simulink model "K_linearLUB"  (R2016a)
settings: Solver=VariableStepAuto  StartTime=0.0  StopTime=1000.0  RelTol=1e-3
undefined symbols (not defined in the file): A, AKL, B, BL, C, CO, D, DO, K, X0
settings Model: Creator=kp  LastModifiedBy=kp

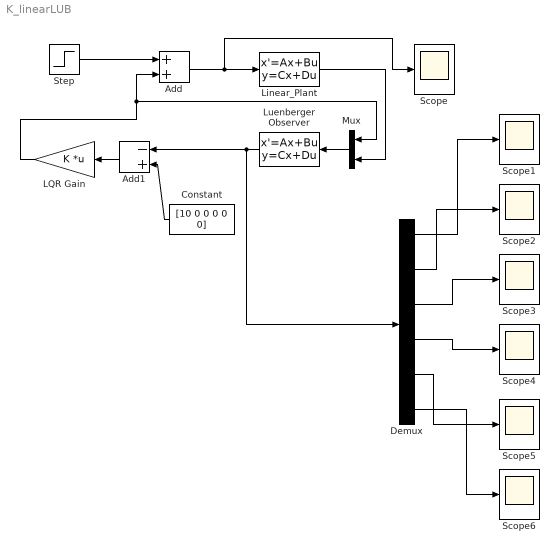
== system K_linearLUB ==
  Add : Sum
  Add1 : Sum  Inputs=-+
  Constant : Constant  Value=[10 0 0 0 0 0]
  Demux : Demux  Outputs=6
  LQR Gain : Gain  Gain=K  Multiplication=Matrix(K*u)
  Linear_Plant : StateSpace  A=A  B=B  C=C  D=D  X0=X0
  Luenberger Observer : StateSpace  A=AKL  B=BL  C=CO  D=DO  X0=0
  Mux : Mux  Inputs=2
  Scope{,1..6} (7 alike) : Scope
  Step : Step  SampleTime=0
  wires:
  Luenberger Observer/1 -> Add1/1, Demux/1
  Add1/1 -> LQR Gain/1
  Mux/1 -> Luenberger Observer/1
  Step/1 -> Add/1
  Add/1 -> Scope/1, Linear_Plant/1
  LQR Gain/1 -> Mux/1, Add/2
  Constant/1 -> Add1/2
  Linear_Plant/1 -> Mux/2
  Demux/1 -> Scope1/1
  Demux/2 -> Scope2/1
  Demux/3 -> Scope3/1
  Demux/4 -> Scope4/1
  Demux/5 -> Scope5/1
  Demux/6 -> Scope6/1
